simulink model "RC"  (R2020b)
settings: Solver=VariableStepAuto  StartTime=0.0  StopTime=0.1  RelTol=1e-3
settings Model: Creator=Akshata Ashok  LastModifiedBy=Akshata Ashok

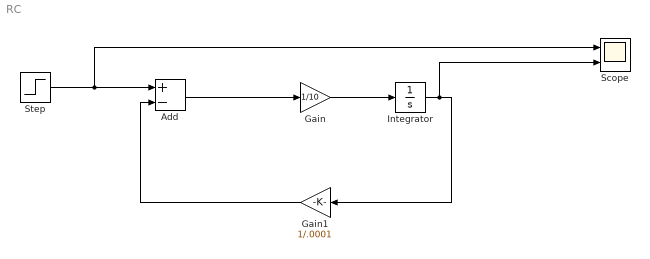
== system RC ==
  Add : Sum  Inputs=+-
  Gain : Gain  Gain=1/10
  Gain1 : Gain  Gain=1/.0001
  Integrator : Integrator  InitialCondition=5  UpperSaturationLimit=5  LowerSaturationLimit=0
  Scope : Scope  NumInputPorts=2
  Step : Step  Before=1  After=0  SampleTime=0.01
  wires:
  Add/1 -> Gain/1
  Gain/1 -> Integrator/1
  Integrator/1 -> Scope/2, Gain1/1
  Gain1/1 -> Add/2
  Step/1 -> Scope/1, Add/1
